simulink model "sim_const"  (R2024b)
settings: Solver=ode45  StartTime=t_0  StopTime=100  FixedStep=dt  RelTol=1e-8
libraries: simulink x1
settings Model: Creator=yevge  LastModifiedBy=Aiden Gaydos
settings DebuggingCC: AlgebraicLoopMsg=error  CheckMatrixSingularityMsg=error

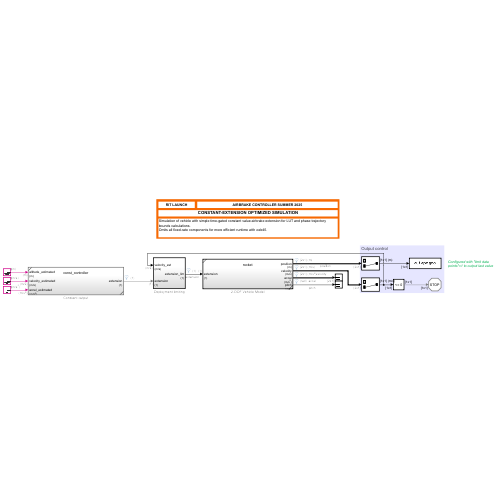
[thumbnail: Simulink's stored preview of the top-level diagram]
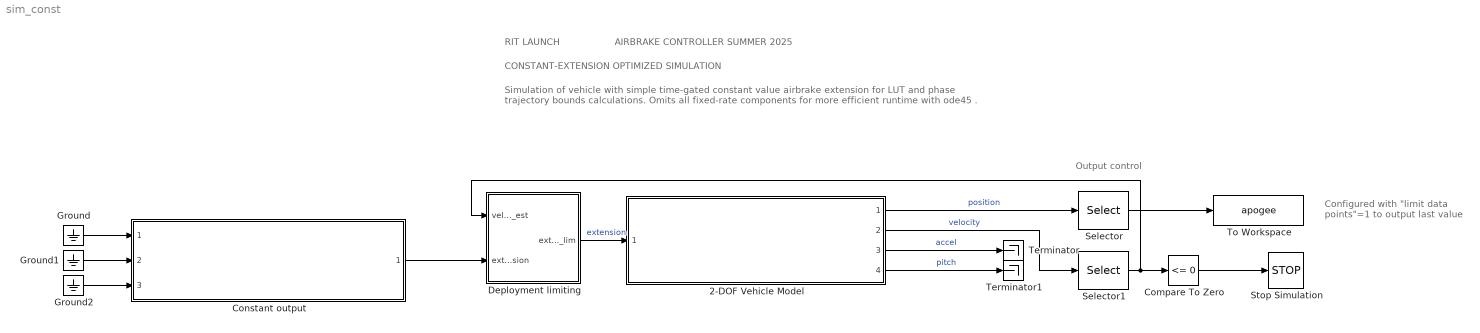
== system sim_const ==
  note: Configured with "limit data points"=1 to output last value
  note: Output control
  note: CONSTANT-EXTENSION OPTIMIZED SIMULATION
  note: RIT LAUNCH
  note: AIRBRAKE CONTROLLER SUMMER 2025
  note: Simulation of vehicle with simple time-gated constant value airbrake extension for LUT and phase trajectory bounds calculations.
      | Omits all fixed-rate components for more efficient runtime with ode45 .
  2-DOF Vehicle Model : Subsystem  ReferencedSubsystem=rocket
  Compare To Zero : simulink/Logic and Bit Operations/Compare To Zero  relop=<=  OutDataTypeStr=boolean
  Constant output : Subsystem  ReferencedSubsystem=const_controller
  Deployment limiting : Subsystem
  Ground : Ground
  Ground1 : Ground
  Ground2 : Ground
  Selector : Selector  InputPortWidth=2  IndexOptions=Index vector (dialog)  Indices=2  OutputSizes=1
  Selector1 : Selector  InputPortWidth=2  IndexOptions=Index vector (dialog)  Indices=2  OutputSizes=1
  Stop Simulation : Stop
  Terminator : Terminator
  Terminator1 : Terminator
  To Workspace : ToWorkspace  VariableName=apogee  SampleTime=-1
      settings: MaxDataPoints=1
  wires:
  Selector/1 -> To Workspace/1
  Selector1/1 -> Deployment limiting/1(velocity_est), Compare To Zero/1
  Compare To Zero/1 -> Stop Simulation/1
  Deployment limiting/1(extension_lim) -> 2-DOF Vehicle Model/1  "extension"
  2-DOF Vehicle Model/1 -> Selector/1  "position"
  2-DOF Vehicle Model/3 -> Terminator/1  "accel"
  2-DOF Vehicle Model/2 -> Selector1/1  "velocity"
  2-DOF Vehicle Model/4 -> Terminator1/1  "pitch"
  Ground/1 -> Constant output/1
  Ground1/1 -> Constant output/2
  Ground2/1 -> Constant output/3
  Constant output/1 -> Deployment limiting/2(extension)

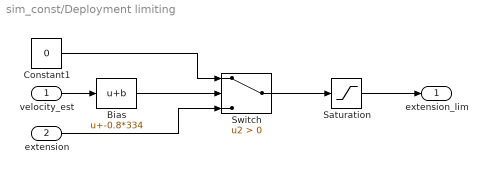
== system sim_const/Deployment limiting ==
  velocity_est : Inport  Unit=m/s  PortDimensions=1
  extension : Inport  Port=2  OutMin=0  OutMax=1  Unit=1  PortDimensions=1
  Bias : Bias  Bias=-0.8*334  SaturateOnIntegerOverflow=off
  Constant1 : Constant  Value=0
  Saturation : Saturate  UpperLimit=1  LowerLimit=0
  Switch : Switch  Criteria=u2 > Threshold  SaturateOnIntegerOverflow=off  InputSameDT=off
  extension_lim : Outport  OutMin=0  OutMax=1  Unit=1  PortDimensions=1
  wires:
  Switch/1 -> Saturation/1
  Constant1/1 -> Switch/1
  extension/1 -> Switch/3
  velocity_est/1 -> Bias/1
  Bias/1 -> Switch/2
  Saturation/1 -> extension_lim/1
